simulink library "pixhawk_slib_adv"  (R2017b)
settings: Solver=ode45  StartTime=0.0  StopTime=10.0  RelTol=1e-3
undefined symbols (not defined in the file or in its folder): Earth, earthRadius, ModelInit_AngEuler, ModelInit_PosE, ModelInit_RateB, ModelInit_RPM, ModelInit_VelB, ModelParam_envAltitude, ModelParam_GPSLatLong, ModelParam_motorCr, ModelParam_motorJm, ModelParam_motorT, ModelParam_motorWb, ModelParam_noisePowerIMU, ModelParam_rotorCm, ModelParam_rotorCt, ModelParam_uavCCm, ModelParam_uavCd, ModelParam_uavDearo, ModelParam_uavJ, ModelParam_uavMass, ModelParam_uavR, ModelParam_uavType, Receive, Send, WGS84
libraries: etargetslib x11, dspnetwork x9, simulink x8, sharedtransform x5, aerolibtransform2 x4, aerolibutil x4, pixhawk_slib_adv x3, aerolibfltsims x3, shared6dof x1, aerolibobsolete x1, aerolibasang x1, aerolibatmos2 x1
(part 3 of 3)

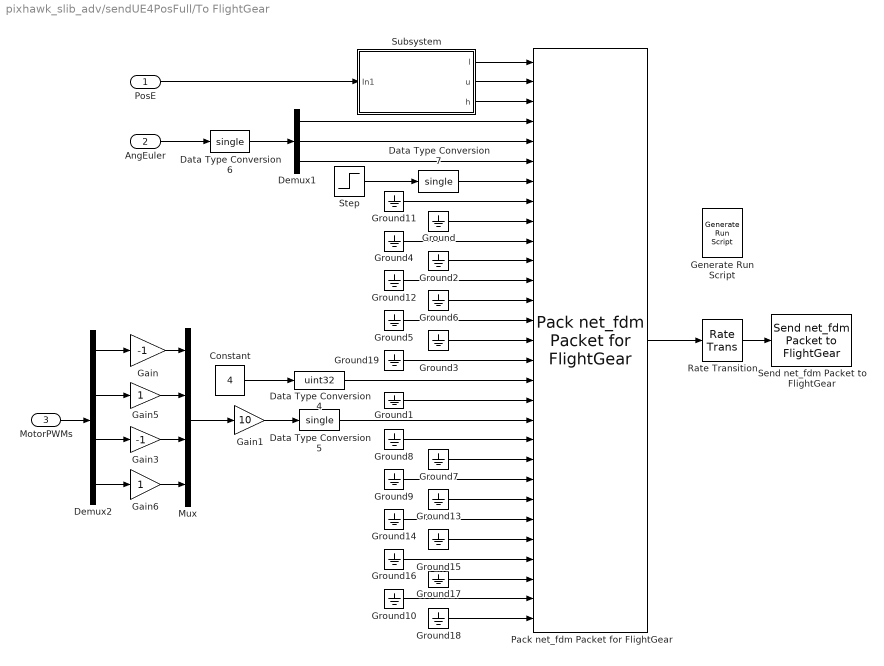
== system pixhawk_slib_adv/sendUE4PosFull/To FlightGear ==
  PosE : Inport
  AngEuler : Inport  Port=2
  MotorPWMs : Inport  Port=3
  Constant : Constant  Value=4
  Data Type Conversion4 : DataTypeConversion  OutDataTypeStr=uint32
  Data Type Conversion5 : DataTypeConversion  OutDataTypeStr=single
  Data Type Conversion6 : DataTypeConversion  OutDataTypeStr=single
  Data Type Conversion7 : DataTypeConversion  OutDataTypeStr=single
  Demux1 : Demux  Outputs=3
  Demux2 : Demux
  Gain : Gain  Gain=-1
  Gain1 : Gain  Gain=10
  Gain3 : Gain  Gain=-1
  Gain5 : Gain
  Gain6 : Gain
  Generate Run Script : aerolibfltsims/Generate Run Script  OutputFileName=runfg_myownUAV.bat  FlightGearBaseDirectory=C:\Program Files\FlightGear 2016.1.2  GeometryModelName=myownUAV  DestinationPort=5502  OriginAddress=127.0.0.1  OriginPort=5505  LocalAddress=127.0.0.1  AirportId=KSFO  RunwayId=10L  InitialAltitude=0  InitialHeading=0  OffsetDistance=0  OffsetAzimuth=0  GenerateFile=off  Architecture=Default  dataFlow=Send-Receive
  Ground{,1..19} (20 alike) : Ground
  Mux : Mux
  Pack net_fdm Packet for FlightGear : aerolibfltsims/Pack net_fdm Packet for FlightGear  FlightGearVersion=v2016.1  ShowPositionAttitudeInputs=on  ShowVelocityAccelerationInputs=off  ShowControlSurfacePositionInputs=on  ShowEngineFuelInputs=on  ShowLandingGearInputs=off  ShowEnvironmentInputs=off  SampleTime=0.01
      settings: SourceProductName=Aerospace Blockset  SourceProductBaseCode=AE
  Rate Transition : RateTransition
  Send net_fdm Packet to FlightGear : aerolibfltsims/Send net_fdm Packet to FlightGear  DestinationIpAddress=127.0.0.1  DestinationPort=5502  LocalIpPort=-1  varLen=off  SampleTime=0.005
      settings: SourceProductName=Aerospace Blockset  SourceProductBaseCode=AE
  Step : Step  Time=0  SampleTime=0
  Subsystem : Subsystem
  wires:
  Gain1/1 -> Data Type Conversion5/1
  Data Type Conversion6/1 -> Demux1/1
  Demux1/3 -> Pack net_fdm Packet for FlightGear/6
  Demux1/2 -> Pack net_fdm Packet for FlightGear/5
  Demux1/1 -> Pack net_fdm Packet for FlightGear/4
  Ground19/1 -> Pack net_fdm Packet for FlightGear/16
  Subsystem/3(h) -> Pack net_fdm Packet for FlightGear/3
  Subsystem/2(u) -> Pack net_fdm Packet for FlightGear/2
  Subsystem/1("l ") -> Pack net_fdm Packet for FlightGear/1
  PosE/1 -> Subsystem/1(In1)
  Rate Transition/1 -> Send net_fdm Packet to FlightGear/1
  Gain6/1 -> Mux/4
  Demux2/4 -> Gain6/1
  Gain5/1 -> Mux/2
  Demux2/2 -> Gain5/1
  Gain3/1 -> Mux/3
  Gain/1 -> Mux/1
  Demux2/3 -> Gain3/1
  Demux2/1 -> Gain/1
  Mux/1 -> Gain1/1
  MotorPWMs/1 -> Demux2/1
  AngEuler/1 -> Data Type Conversion6/1
  Ground12/1 -> Pack net_fdm Packet for FlightGear/12
  Ground2/1 -> Pack net_fdm Packet for FlightGear/11
  Data Type Conversion5/1 -> Pack net_fdm Packet for FlightGear/19
  Constant/1 -> Data Type Conversion4/1
  Ground11/1 -> Pack net_fdm Packet for FlightGear/8
  Ground4/1 -> Pack net_fdm Packet for FlightGear/10
  Ground6/1 -> Pack net_fdm Packet for FlightGear/13
  Ground5/1 -> Pack net_fdm Packet for FlightGear/14
  Ground3/1 -> Pack net_fdm Packet for FlightGear/15
  Ground1/1 -> Pack net_fdm Packet for FlightGear/18
  Data Type Conversion4/1 -> Pack net_fdm Packet for FlightGear/17
  Step/1 -> Data Type Conversion7/1
  Ground18/1 -> Pack net_fdm Packet for FlightGear/29
  Ground10/1 -> Pack net_fdm Packet for FlightGear/28
  Ground17/1 -> Pack net_fdm Packet for FlightGear/27
  Ground16/1 -> Pack net_fdm Packet for FlightGear/26
  Ground15/1 -> Pack net_fdm Packet for FlightGear/25
  Ground14/1 -> Pack net_fdm Packet for FlightGear/24
  Ground13/1 -> Pack net_fdm Packet for FlightGear/23
  Ground9/1 -> Pack net_fdm Packet for FlightGear/22
  Ground7/1 -> Pack net_fdm Packet for FlightGear/21
  Ground/1 -> Pack net_fdm Packet for FlightGear/9
  Ground8/1 -> Pack net_fdm Packet for FlightGear/20
  Data Type Conversion7/1 -> Pack net_fdm Packet for FlightGear/7
  Pack net_fdm Packet for FlightGear/1 -> Rate Transition/1

== system pixhawk_slib_adv/CopterMotorModel/MotorNonlinearDynamic1/Motor_Dynamics ==
  motor_rate_d : Inport
  ModelInit_RPM : Inport  Port=2
  motorT : Inport  Port=3
  Add : Sum  Inputs=+-
  Divide : Product  Inputs=*/
  Integrator : Integrator  InitialConditionSource=external
  motor_rate_act : Outport
  wires:
  motorT/1 -> Divide/2
  Integrator/1 -> Add/2, motor_rate_act/1  "x"
  Divide/1 -> Integrator/1  "drate/dt"
  motor_rate_d/1 -> Add/1
  ModelInit_RPM/1 -> Integrator/2
  Add/1 -> Divide/1

== system pixhawk_slib_adv/CopterMotorModel/MotorNonlinearDynamic2/Motor_Dynamics ==
  motor_rate_d : Inport
  ModelInit_RPM : Inport  Port=2
  motorT : Inport  Port=3
  Add : Sum  Inputs=+-
  Divide : Product  Inputs=*/
  Integrator : Integrator  InitialConditionSource=external
  motor_rate_act : Outport
  wires:
  Add/1 -> Divide/1
  ModelInit_RPM/1 -> Integrator/2
  motor_rate_d/1 -> Add/1
  Divide/1 -> Integrator/1  "drate/dt"
  Integrator/1 -> motor_rate_act/1, Add/2  "x"
  motorT/1 -> Divide/2

== system pixhawk_slib_adv/CopterMotorModel/MotorNonlinearDynamic3/Motor_Dynamics ==
  motor_rate_d : Inport
  ModelInit_RPM : Inport  Port=2
  motorT : Inport  Port=3
  Add : Sum  Inputs=+-
  Divide : Product  Inputs=*/
  Integrator : Integrator  InitialConditionSource=external
  motor_rate_act : Outport
  wires:
  motorT/1 -> Divide/2
  Integrator/1 -> Add/2, motor_rate_act/1  "x"
  Divide/1 -> Integrator/1  "drate/dt"
  motor_rate_d/1 -> Add/1
  ModelInit_RPM/1 -> Integrator/2
  Add/1 -> Divide/1

== system pixhawk_slib_adv/CopterMotorModel/MotorNonlinearDynamic4/Motor_Dynamics ==
  motor_rate_d : Inport
  ModelInit_RPM : Inport  Port=2
  motorT : Inport  Port=3
  Add : Sum  Inputs=+-
  Divide : Product  Inputs=*/
  Integrator : Integrator  InitialConditionSource=external
  motor_rate_act : Outport
  wires:
  Add/1 -> Divide/1
  ModelInit_RPM/1 -> Integrator/2
  motor_rate_d/1 -> Add/1
  Divide/1 -> Integrator/1  "drate/dt"
  Integrator/1 -> motor_rate_act/1, Add/2  "x"
  motorT/1 -> Divide/2

== system pixhawk_slib_adv/CopterMotorModel/MotorNonlinearDynamic5/Motor_Dynamics ==
  motor_rate_d : Inport
  ModelInit_RPM : Inport  Port=2
  motorT : Inport  Port=3
  Add : Sum  Inputs=+-
  Divide : Product  Inputs=*/
  Integrator : Integrator  InitialConditionSource=external
  motor_rate_act : Outport
  wires:
  motorT/1 -> Divide/2
  Integrator/1 -> Add/2, motor_rate_act/1  "x"
  Divide/1 -> Integrator/1  "drate/dt"
  motor_rate_d/1 -> Add/1
  ModelInit_RPM/1 -> Integrator/2
  Add/1 -> Divide/1

== system pixhawk_slib_adv/CopterMotorModel/MotorNonlinearDynamic6/Motor_Dynamics ==
  motor_rate_d : Inport
  ModelInit_RPM : Inport  Port=2
  motorT : Inport  Port=3
  Add : Sum  Inputs=+-
  Divide : Product  Inputs=*/
  Integrator : Integrator  InitialConditionSource=external
  motor_rate_act : Outport
  wires:
  Add/1 -> Divide/1
  ModelInit_RPM/1 -> Integrator/2
  motor_rate_d/1 -> Add/1
  Divide/1 -> Integrator/1  "drate/dt"
  Integrator/1 -> motor_rate_act/1, Add/2  "x"
  motorT/1 -> Divide/2

== system pixhawk_slib_adv/CopterMotorModel/MotorNonlinearDynamic7/Motor_Dynamics ==
  motor_rate_d : Inport
  ModelInit_RPM : Inport  Port=2
  motorT : Inport  Port=3
  Add : Sum  Inputs=+-
  Divide : Product  Inputs=*/
  Integrator : Integrator  InitialConditionSource=external
  motor_rate_act : Outport
  wires:
  motorT/1 -> Divide/2
  Integrator/1 -> Add/2, motor_rate_act/1  "x"
  Divide/1 -> Integrator/1  "drate/dt"
  motor_rate_d/1 -> Add/1
  ModelInit_RPM/1 -> Integrator/2
  Add/1 -> Divide/1

== system pixhawk_slib_adv/CopterMotorModel/MotorNonlinearDynamic8/Motor_Dynamics ==
  motor_rate_d : Inport
  ModelInit_RPM : Inport  Port=2
  motorT : Inport  Port=3
  Add : Sum  Inputs=+-
  Divide : Product  Inputs=*/
  Integrator : Integrator  InitialConditionSource=external
  motor_rate_act : Outport
  wires:
  Add/1 -> Divide/1
  ModelInit_RPM/1 -> Integrator/2
  motor_rate_d/1 -> Add/1
  Divide/1 -> Integrator/1  "drate/dt"
  Integrator/1 -> motor_rate_act/1, Add/2  "x"
  motorT/1 -> Divide/2

== system pixhawk_slib_adv/SensorOutput/HILGPSModel/GyroNoiseSwitch1 ==
  In1 : Inport
  Constant1 : Constant  Value=Param_GlobalNoiseGainSwitch
  Constant2 : Constant  Value=0.3
  Gain2 : Gain  Gain=0.7
  Product4 : Product
  Sum : Sum  Inputs=|++
  Out1 : Outport
  wires:
  Sum/1 -> Product4/2
  Product4/1 -> Out1/1
  Gain2/1 -> Sum/1
  In1/1 -> Product4/1
  Constant1/1 -> Gain2/1
  Constant2/1 -> Sum/2

== system pixhawk_slib_adv/SensorOutput/HILGPSModel/NoiseFilter1 ==
  In1 : Inport
  Demux : Demux  Outputs=3
  Mux1 : Mux  Inputs=3
  Transfer Fcn1 : TransferFcn  Denominator=[0.05 1]
  Transfer Fcn2 : TransferFcn  Denominator=[0.05 1]
  Transfer Fcn4 : TransferFcn  Denominator=[0.05 1]
  Out1 : Outport
  wires:
  Mux1/1 -> Out1/1
  In1/1 -> Demux/1
  Demux/3 -> Transfer Fcn2/1
  Transfer Fcn4/1 -> Mux1/1
  Transfer Fcn2/1 -> Mux1/3
  Demux/1 -> Transfer Fcn4/1
  Transfer Fcn1/1 -> Mux1/2
  Demux/2 -> Transfer Fcn1/1

== system pixhawk_slib_adv/SensorOutput/HILGPSModel/Subsystem ==
  u : Inport
  Constant : Constant  Value=0
  Constant1 : Constant  Value=360
  Demux1 : Demux  Outputs=3
  Product : Product
  Product1 : Product
  Sqrt : Sqrt  SaturateOnIntegerOverflow=on
  Sum1 : Sum  Inputs=|++
  Sum4 : Sum  Inputs=|++
  Switch : Switch  Threshold=1
  Switch1 : Switch
  Terminator : Terminator
  Trigonometric Function : Trigonometry  Operator=atan2
  v : Outport
  cot : Outport  Port=2
  wires:
  Demux1/2 -> Trigonometric Function/2, Product1/2, Product1/1
  Product/1 -> Sum4/1
  u/1 -> Demux1/1
  Switch/1 -> Sum1/1, Switch1/1, Switch1/2
  Product1/1 -> Sum4/2
  Demux1/3 -> Terminator/1
  Sqrt/1 -> v/1, Switch/2
  Constant/1 -> Switch/3
  Trigonometric Function/1 -> Switch/1
  Sum4/1 -> Sqrt/1
  Demux1/1 -> Trigonometric Function/1, Product/1, Product/2
  Constant1/1 -> Sum1/2
  Sum1/1 -> Switch1/3
  Switch1/1 -> cot/1

== system pixhawk_slib_adv/SensorOutput/HILSensorMavModel/GyroNoiseSwitch0 ==
  In1 : Inport
  Constant1 : Constant  Value=Param_GlobalNoiseGainSwitch
  Constant2 : Constant  Value=0.2
  Gain2 : Gain  Gain=0.8
  Product4 : Product
  Sum : Sum  Inputs=|++
  Out1 : Outport
  wires:
  Sum/1 -> Product4/2
  Product4/1 -> Out1/1
  Gain2/1 -> Sum/1
  In1/1 -> Product4/1
  Constant1/1 -> Gain2/1
  Constant2/1 -> Sum/2

== system pixhawk_slib_adv/SensorOutput/HILSensorMavModel/GyroNoiseSwitch1 ==
  In1 : Inport
  Constant1 : Constant  Value=Param_GlobalNoiseGainSwitch
  Constant2 : Constant  Value=0.2
  Gain2 : Gain  Gain=0.8
  Product4 : Product
  Sum : Sum  Inputs=|++
  Out1 : Outport
  wires:
  Sum/1 -> Product4/2
  Product4/1 -> Out1/1
  Gain2/1 -> Sum/1
  In1/1 -> Product4/1
  Constant1/1 -> Gain2/1
  Constant2/1 -> Sum/2

== system pixhawk_slib_adv/SensorOutput/HILSensorMavModel/GyroNoiseSwitch2 ==
  In1 : Inport
  Constant1 : Constant  Value=Param_GlobalNoiseGainSwitch
  Constant2 : Constant  Value=0.2
  Gain2 : Gain  Gain=0.8
  Product4 : Product
  Sum : Sum  Inputs=|++
  Out1 : Outport
  wires:
  Sum/1 -> Product4/2
  Product4/1 -> Out1/1
  Gain2/1 -> Sum/1
  In1/1 -> Product4/1
  Constant1/1 -> Gain2/1
  Constant2/1 -> Sum/2

== system pixhawk_slib_adv/SensorOutput/HILSensorMavModel/GyroNoiseSwitch3 ==
  In1 : Inport
  Constant1 : Constant  Value=Param_GlobalNoiseGainSwitch
  Constant2 : Constant  Value=0.3
  Gain2 : Gain  Gain=0.7
  Product4 : Product
  Sum : Sum  Inputs=|++
  Out1 : Outport
  wires:
  Sum/1 -> Product4/2
  Product4/1 -> Out1/1
  Gain2/1 -> Sum/1
  In1/1 -> Product4/1
  Constant1/1 -> Gain2/1
  Constant2/1 -> Sum/2

== system pixhawk_slib_adv/SensorOutput/HILSensorMavModel/GyroNoiseSwitch4 ==
  In1 : Inport
  Constant1 : Constant  Value=Param_GlobalNoiseGainSwitch
  Constant2 : Constant  Value=0.3
  Gain2 : Gain  Gain=0.7
  Product4 : Product
  Sum : Sum  Inputs=|++
  Out1 : Outport
  wires:
  Sum/1 -> Product4/2
  Product4/1 -> Out1/1
  Gain2/1 -> Sum/1
  In1/1 -> Product4/1
  Constant1/1 -> Gain2/1
  Constant2/1 -> Sum/2

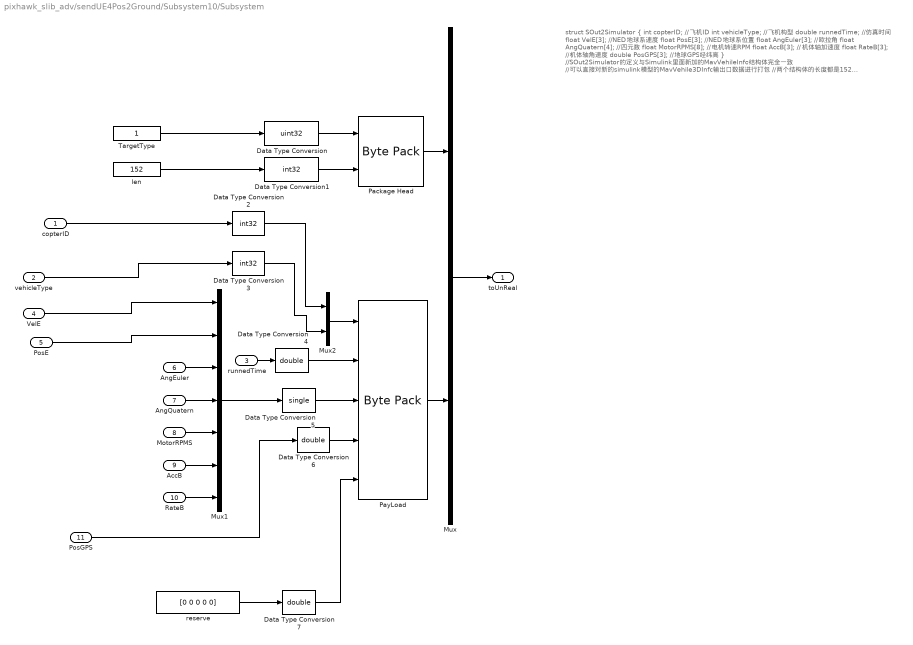
== system pixhawk_slib_adv/sendUE4Pos2Ground/Subsystem10/Subsystem ==
  note: struct SOut2Simulator
      | {
      | int copterID; //飞机ID
      | int vehicleType; //飞机构型
      | double runnedTime; //仿真时间
      | float VelE[3]; //NED地球系速度
      | float PosE[3]; //NED地球系位置
      | float AngEuler[3]; //欧拉角
      | float AngQuatern[4]; //四元数
      | float MotorRPMS[8]; //电机转速RPM
      | float AccB[3]; //机体轴加速度
      | float RateB[3]; //机体轴角速度
      | double PosGPS[3]; //地球GPS经纬高
      | }
      |
      | //SOut2Simulator的定义与Simulink里面新加的MavVehileInfo结构体完全一致
      | //可以直接对新的simulink模型的MavVehile3DInfo输出口数据进行打包
      | //两个结构体的长度都是152
      | sizeof(SOut2Simulator) = sizeof(MavVehileInfo) = 152
      |
      | 打包封装的结构体为
      | typedef struct _netDataShort
      | {
      | TargetType tg; //这里目前随便填，写1即可 uint32
      | int len; //这个长度为传输结构体长度，目前是152
      | char payload[192]; //这里面前152位存放了SOut2Simulator结构体数据，后面的40位保留
      | }netDataShort;
      |
      | //UDP包的总长度为200
      | sizeof(netDataShort) = 200
      |
      | //发送的UDP端口号为：20010
  copterID : Inport  PortDimensions=1
  vehicleType : Inport  Port=2  PortDimensions=1
  runnedTime : Inport  Port=3  PortDimensions=1
  "VelE " : Inport  Port=4  PortDimensions=3
  PosE : Inport  Port=5  PortDimensions=3
  AngEuler : Inport  Port=6  PortDimensions=3
  AngQuatern : Inport  Port=7  PortDimensions=4
  MotorRPMS : Inport  Port=8  PortDimensions=8
  AccB : Inport  Port=9  PortDimensions=3
  RateB : Inport  Port=10  PortDimensions=3
  PosGPS : Inport  Port=11  PortDimensions=3
  Data Type Conversion : DataTypeConversion  OutDataTypeStr=uint32
  Data Type Conversion1 : DataTypeConversion  OutDataTypeStr=int32
  Data Type Conversion2 : DataTypeConversion  OutDataTypeStr=int32
  Data Type Conversion3 : DataTypeConversion  OutDataTypeStr=int32
  Data Type Conversion4 : DataTypeConversion  OutDataTypeStr=double
  Data Type Conversion5 : DataTypeConversion  OutDataTypeStr=single
  Data Type Conversion6 : DataTypeConversion  OutDataTypeStr=double
  Data Type Conversion7 : DataTypeConversion  OutDataTypeStr=double
  Mux : Mux  Inputs=2
  Mux1 : Mux  Inputs=7
  Mux2 : Mux  Inputs=2
  Package Head : etargetslib/Byte Pack  datatypes={'uint32','int32'}  byteAlign=4
  PayLoad : etargetslib/Byte Pack  datatypes={'int32','double','single','double','double'}  byteAlign=8
  TargetType : Constant  OutDataTypeStr=Inherit: Inherit via back propagation
  len : Constant  Value=152  OutDataTypeStr=Inherit: Inherit via back propagation
  reserve : Constant  Value=[0 0 0 0 0]  OutDataTypeStr=double
  toUnReal : Outport
  wires:
  runnedTime/1 -> Data Type Conversion4/1
  RateB/1 -> Mux1/7
  PayLoad/1 -> Mux/2
  "VelE "/1 -> Mux1/1
  Mux1/1 -> Data Type Conversion5/1
  PosGPS/1 -> Data Type Conversion6/1
  Package Head/1 -> Mux/1
  AccB/1 -> Mux1/6
  Mux/1 -> toUnReal/1
  MotorRPMS/1 -> Mux1/5
  AngQuatern/1 -> Mux1/4
  copterID/1 -> Data Type Conversion2/1
  len/1 -> Data Type Conversion1/1
  vehicleType/1 -> Data Type Conversion3/1
  PosE/1 -> Mux1/2
  TargetType/1 -> Data Type Conversion/1
  reserve/1 -> Data Type Conversion7/1
  Mux2/1 -> PayLoad/1
  AngEuler/1 -> Mux1/3
  Data Type Conversion5/1 -> PayLoad/3
  Data Type Conversion2/1 -> Mux2/1
  Data Type Conversion1/1 -> Package Head/2
  Data Type Conversion6/1 -> PayLoad/4
  Data Type Conversion/1 -> Package Head/1
  Data Type Conversion3/1 -> Mux2/2
  Data Type Conversion4/1 -> PayLoad/2
  Data Type Conversion7/1 -> PayLoad/5

== system pixhawk_slib_adv/sendUE4PosFull/To FlightGear/Subsystem ==
  In1 : Inport
  Constant1 : Constant  Value=5  VectorParams1D=off
  Constant2 : Constant  Value=-2.1361  VectorParams1D=off
  Constant3 : Constant  Value=0.65673  VectorParams1D=off
  Demux : Demux  Outputs=3
  Gain1 : Gain  Gain=10/earthRadius
  Gain2 : Gain  Gain=10/earthRadius
  Gain4 : Gain
  Gain8 : Gain  Gain=-10
  Sum10 : Sum  Inputs=|++
  Sum8 : Sum  Inputs=|++
  Sum9 : Sum  Inputs=|++
  "l " : Outport
  u : Outport  Port=2
  h : Outport  Port=3
  wires:
  Sum8/1 -> "l "/1
  In1/1 -> Demux/1
  Sum9/1 -> u/1
  Sum10/1 -> h/1
  Gain4/1 -> Gain2/1
  Demux/2 -> Gain1/1
  Gain8/1 -> Sum10/1
  Gain1/1 -> Sum8/1
  Gain2/1 -> Sum9/1
  Constant2/1 -> Sum8/2
  Demux/3 -> Gain8/1
  Demux/1 -> Gain4/1
  Constant1/1 -> Sum10/2
  Constant3/1 -> Sum9/2

== matlab function pixhawk_slib_adv/getTerrainAltData ==
  data: x input; z output; y input
function z = fcn(x,y)
z=getTerrainAltData(x,y);

== matlab function pixhawk_slib_adv/CopterForceModel/Propeller Model old Version ==
  data: uavType input; MotorRads input; R input; Fb output; Mb output; Cm input; Ct input; Jm input; wb input
function [Fb,Mb] = fcn(uavType,MotorRads,R,Cm,Ct,Jm,wb)
% This is control effectiveness model, where Fb is the force produced by motors, Mb is
% the moment produced by motors, and Fd is the resistance produced by the air.
% The gyroscopic torque is not considered here.

% -1: anticlockwise, 1: clockwise 
TypeMotorDirMatrix=[...
    [-1 -1 -1 0 0 0 0 0];... % Tri 3*1 X
    [1 1 1 0 0 0 0 0];...    % Tri 3*1 +
    [-1 -1 1 1 0 0 0 0];... % Quad 4*1 X
    [-1 -1 1 1 0 0 0 0];... % Quad 4*1 +
    [1 -1 1 -1 -1 1 0 0];... % Hex 6*1 X
    [1 -1 1 -1 -1 1 0 0];... % Hex 6*1 +
    [1 -1 1 -1 1 -1 0 0];... % HexCoa 3*2
    [1 1 -1 -1 -1 -1 1 1];... % Oct 8*1 X
    [1 1 -1 -1 -1 -1 1 1];... % Oct 8*1 +
    [-1 1 -1 1 -1 1 -1 1];... % OctCoa 4*2 X
];

TypeMotorAngMatrix=[...
    [pi/3 pi -pi/3 0 0 0 0 0];...
    [pi/3 pi -pi/3 0 0 0 0 0];...
    [pi/4 pi/4+pi pi/4+3*pi/2 pi/4+pi/2 0 0 0 0];...
    [pi/2 3*pi/2 0 pi 0 0 0 0];...
    [pi/2 3/2*pi 3/2*pi+pi/3 pi/2+pi/3 pi/2-pi/3 3/2*pi-pi/3 0 0];...
    [0 pi pi+pi/3 pi/3 -pi/3 pi-pi/3 0 0];...
    [pi/3 pi/3 pi pi -pi/3 -pi/3 0 0];...
    [pi/8 pi+pi/8 pi/8+pi/4 pi-pi/8 -pi/8 3/2*pi-pi/8 3/2*pi+pi/8 pi/2+pi/8];...
    [0 pi pi/4 3/4*pi -pi/4 pi+pi/4 3/2*pi pi/2];...
    [pi/4 -pi/4 pi+pi/4 pi-pi/4 -pi/4 pi/4 pi-pi/4 pi+pi/4];...
];

TypeMotorNonVector=int8([3;3;4;4;6;6;6;8;8;8]);

Mb = [0;0;0];
Fb = [0;0;0];
P=wb(1);Q=wb(2);

if uavType==50
    
    Fb(1)=MotorRads(1)+MotorRads(3);
    Mb(3)=MotorRads(1)*0.1-MotorRads(3)*0.1;
    
    return;
end


if uavType<0||uavType>length(TypeMotorNonVector)
    uavType=int16(1);
end

TypeMotorDirVector=TypeMotorDirMatrix(uavType,:);
TypeMotorAngVector=TypeMotorAngMatrix(uavType,:);

for i=1:TypeMotorNonVector(uavType)
    propAng = TypeMotorAngVector(i);
    propdir = TypeMotorDirVector(i);
    PropT = Ct*MotorRads(i)*MotorRads(i);
    PropM = Cm*MotorRads(i)*MotorRads(i);
    
    %Thrust -> Moment
    Mb=Mb+[-R*sin(propAng)*PropT;R*cos(propAng)*PropT;-PropM*propdir];
    
    %gyroscopic moment
    Mb=Mb+[Q*Jm*MotorRads(i)*propdir;-P*Jm*MotorRads(i)*propdir;0];
    
    Fb=Fb+[0;0;-PropT];
end

 
end

== matlab function pixhawk_slib_adv/PlaneGroundModel/Ground Model ==
  settings: updateMethod=DISCRETE
  data: mg input; wb input; Xe input; F1 output; Ve input; M1 output; Quet input; terrainZ input
function [F1,M1] = fcn(mg,wb,Xe,Ve,Quet,terrainZ)
% This is a ground model that can provides reaction force and reaction torque

% persistent z0;
% if isempty(z0)
%      z0=0;
% end
terrainZ=terrainZ(1)
persistent takeoffFlag;
if isempty(takeoffFlag)
     takeoffFlag=int8(0);
end

persistent landFlag;
if isempty(landFlag)
     landFlag=int8(1);
end


z=Xe(3)-terrainZ;

 if (z<-0.3)&&(Ve(3)<-0.1)&&(takeoffFlag<0.5)
    takeoffFlag=int8(1);
    landFlag=int8(0);
 end
 
 if (z>-0.05)&&(Ve(3)>0.1)&&(landFlag<0.5)
    landFlag=int8(1);
    takeoffFlag=int8(0);
    %z0=terrainZ;
 end

takeoff = takeoffFlag;
landed = landFlag;


F1=[0;0;0];
M1=[0;0;0];

if z>=0
%     if z>=0.3
%         if Ve(3)>=5
%             F1(3)=-mg(3)-1000*Ve(3);
%         else
%             F1(3)=-mg(3)-500*z-100*Ve(3);  
%         end
%     elseif z>=0.1
%         if Ve(3)>=2
%             F1(3)=-mg(3)-100*Ve(3);
%         else
%             F1(3)=-mg(3)-50*z-100*Ve(3);  
%         end
%     else
%          if Ve(3)>=1
%             F1(3)=-mg(3)-50*Ve(3);
%         else
%             F1(3)=-mg(3)-5*z-50*Ve(3);  
%         end       
%     end
    if z<0.05
         F1(3)=-mg(3)-10*Ve(3); 
    elseif z<0.1
        F1(3)=-mg(3)-0.5*z-20*Ve(3); 
    else
         F1(3)=-mg(3)-1*z-50*Ve(3); 
    end

    
    F1(1)=-2*Ve(1);
    F1(2)=-50*Ve(2);
    M1=-20*[Quet(2);Quet(3);Quet(4)]-5*wb;
    M1 = M1 * abs(mg(3))*0.0333;
end

== matlab function pixhawk_slib_adv/LoadPngData ==
  data: pngMapName input
function fcn(pngMapName)

LoadPngData(pngMapName);

== matlab function pixhawk_slib_adv/CopterGroundModel/Ground Model ==
  settings: updateMethod=DISCRETE
  data: mg input; wb input; Xe input; F1 output; Ve input; M1 output; Quet input; TerrainIn input
function [F1,M1] = fcn(mg,wb,Xe,Ve,Quet,TerrainIn)
% This is a ground model that can provides reaction force and reaction torque

terrainZ=TerrainIn(1); %暂时提取高程数据

% persistent z0;
% if isempty(z0)
%      z0=0;
% end

persistent takeoffFlag;
if isempty(takeoffFlag)
     takeoffFlag=int8(0);
end

persistent landFlag;
if isempty(landFlag)
     landFlag=int8(1);
end


z=Xe(3)-terrainZ;

 if (z<-0.3)&&(Ve(3)<-0.1)&&(takeoffFlag<0.5)
    takeoffFlag=int8(1);
    landFlag=int8(0);
 end
 
 if (z>-0.05)&&(Ve(3)>0.1)&&(landFlag<0.5)
    landFlag=int8(1);
    takeoffFlag=int8(0);
    %z0=terrainZ;
 end

takeoff = takeoffFlag;
landed = landFlag;


F1=[0;0;0];
M1=[0;0;0];

if z>=0

    if z<0.01
         F1(3)=-mg(3)-200*z-200*Ve(3); 
    elseif z<0.03
        F1(3)=-mg(3)-500*z-500*Ve(3); 
    else
         F1(3)=-mg(3)-1000*z-1000*Ve(3); 
    end

    
    F1(1)=-50*Ve(1);
    F1(2)=-50*Ve(2);
    M1=-20*[Quet(2);Quet(3);Quet(4)]-5*wb;
    M1 = M1 * abs(mg(3))*0.0333;
end

== matlab function pixhawk_slib_adv/sendUE4CMD ==
  data: x input
function RflySendUE4CMD(x)
% x y z为设置相机的位置，单位m，北东地
%roll pitch yaw为设置相机方向，单位度

if ~exist('x','var')
   x='RflyChangeMapbyName Grasslands';
end

out = uint8(x);
len=length(out);
yy=[out,uint8(zeros(1,52-len))];
yy=[typecast(int32(1234567890),'uint8'),yy];
u=udp('255.255.255.255','RemotePort',20010);
fopen(u);
fwrite(u,yy);
fclose(u);
delete(u)

end

== matlab function pixhawk_slib_adv/RflyCameraPosAng ==
  data: x input; y input; z input; roll input; pitch input; yaw input
function RflyCameraPosAng(x,y,z,roll,pitch,yaw)
% x y z为设置相机的位置，单位m，北东地
%roll pitch yaw为设置相机方向，单位度

if ~exist('x','var')
   x=0;
end


if ~exist('y','var')
   y=0;
end

if ~exist('z','var')
   z=0;
end

if ~exist('roll','var')
   roll=0;
end

if ~exist('pitch','var')
   pitch=0;
end


if ~exist('yaw','var')
   yaw=0;
end

out = uint8(['RflyCameraPosAng ',num2str(x),' ',num2str(y),' ',num2str(z),' ',num2str(roll),' ',num2str(pitch),' ',num2str(yaw)]);
len=length(out);
yy=[out,uint8(zeros(1,52-len))];
yy=[typecast(int32(1234567890),'uint8'),yy];
u=udp('255.255.255.255','RemotePort',20010);
fopen(u);
fwrite(u,yy);
fclose(u);
delete(u)
%u3=udp('127.0.0.1','RemotePort',8848,'LocalPort',8850);%同上

end

== matlab function pixhawk_slib_adv/RflyChangeMap/MATLAB Function ==
  data: data output; input input
function data = ChangeMap(input)
    if ischar(input)
        % 通过地图名称修改
        cmd = ['RflyChangeMapbyName ', input];
    elseif isnumeric(input)
        % 通过地图ID修改
        cmd = ['RflyChangeMapbyID ', num2str(input)];
    else
        error('输入必须是字符串或数字');
    end
    
    % 将命令字符串转换为uint8并填充为252长度
    data = [uint8(cmd), uint8(zeros(1, 252 - length(cmd)))]; 
end

== matlab function pixhawk_slib_adv/SensorOutput/HILGPSModel/GenCogVel ==
  data: v output; u input; cot output
function [v,cot] = Ang360(u)
v=norm(u(1:2));

if v < 1
    cot = 0;
else
    cot=atan2d(u(2),u(1));
end
 
if cot<0
    cot=cot+360;
end

== matlab function pixhawk_slib_adv/sendUE4Pos2Ground/getTerrainAltData9 ==
  data: x input; z output; y input
function z = fcn(x,y)
z=getTerrainAltData(x,y);

== matlab function pixhawk_slib_adv/UDP_20100_PX4SilRecv/DataValidation ==
  data: inGPSPos input; outGPSPos output; inGpsVel input; inEulerAng input; outGpsVel output; outEulerAng output; outDataOk output
function [outGPSPos,outGpsVel,outEulerAng,outDataOk] = fcn(inGPSPos,inGpsVel,inEulerAng)

outGPSPos = [0;0;0];
outGpsVel = [0;0;0];
outEulerAng = [0;0;0];
outDataOk = 0;

if(abs(inGPSPos(1))<10000)
    outGPSPos=inGPSPos;
    outGpsVel=inGpsVel;
    outEulerAng = inEulerAng;
    outDataOk = 1;
end

== matlab function pixhawk_slib_adv/UDP_30100_TrueSimRecv/VehicleDataPerse1 ==
  data: Data input; y output double; dataOk output

% //FULL完整模式，输出到RflySim3D的数据
% struct SOut2Simulator {
%     int checksum; // 校验码123456789，必须设定为本值，才会认为是有效数据
%     int copterID;  //飞机ID序号
%     int vehicleType;  //载具样式ID，对应UE的XML中ClassID
%     int reserv; //备用标志位，Int型，将来用于表示碰撞、或大地图等标识
%     float VelE[3];   //速度，北东地，单位米/s
%     float AngEuler[3];  //欧拉角，滚转俯仰偏航，单位弧度
%     float AngQuatern[4]; //姿态四元数向量，w x y z
%     float MotorRPMS[8];  //执行器偏转量或转速，旋翼类对应RPM转每分
%     float AccB[3];       //载具机体FRD坐标系下加速度
%     float RateB[3];      //载具机体FRD坐标系下角速度，pqr，单位rad/s
%     double runnedTime; //时间戳，仿真开始为0时刻。
%     double PosE[3];   //北东地位置，单位米，z向下为正
%     double PosGPS[3];    //载具纬度、经度、高度向量，单位度和米，高度向上为正
% };
% // Python解码标识4i24f7d，数据长度168字节

% 
% 
% len = typecast(Data(5:8), 'int32');
% 
% if len ~= 152
%    return; 
% end
% 
% y = Data(9:160);
% dataOk = 1;

function [y, dataOk] = fcn(Data)
    % Initialize output
    dataOk = 0;

    % Persistent variable to store parsed data
    persistent UIV;
    if isempty(UIV)
        UIV = zeros(35, 1);
    end

    % Calculate length of the received data
    Length = numel(Data);

    % Check if data length matches the expected 168 bytes
    if Length == 168
        % Parse the checksum (first 4 bytes)
        checksum = typecast(Data(1:4), 'int32');
        
        % Verify checksum value
        if checksum == 123456789
            % Define index for parsing
            eIdx = 4 * 4;
            
            % Parse integer values (first 16 bytes)
            intVal = typecast(Data(1:eIdx), 'int32');
            
            % Parse single-precision float values (next 96 bytes)
            floatVal = typecast(Data(eIdx+1:eIdx+24*4), 'single');
            eIdx = eIdx + 24*4;
            
            % Parse double-precision float values (next 56 bytes)
            doubVal = typecast(Data(eIdx+1:eIdx+8*7), 'double');
            
            % Combine all parsed values into the persistent variable UIV
            UIV = [double(intVal); double(floatVal); doubVal];
            dataOk = 1;
        end
    end
    
    % Output the parsed data
    y = UIV;
end

== matlab function pixhawk_slib_adv/UDP_40100_RflyPx4Recv/VehicleDataPerse ==
  data: Data input; y output uint8 size=[48,1]; dataOk output
function [y, dataOk] = fcn(Data)
    % Initialize output
    y = uint8(zeros(48, 1));
    dataOk = 0;

    % Calculate length of the received data
    Length = numel(Data);

    % Check if data length matches the expected 48 bytes
    if Length ~= 48
        return;
    end

    % Parse the checksum (first 4 bytes)
    checksum = typecast(Data(1:4), 'int32');

    % Verify checksum value
    if checksum ~= 1234567898
        return;
    end

    % If checksum is correct, copy data to output
    y = Data(1:48);
    dataOk = 1;
end

== matlab function pixhawk_slib_adv/CopterForceModel/Body AeroCenter ==
  data: Fd output; Md output; wb input; Vb input; Cd input; CCm input; uavDearo input
function [Fd,Md] = fcn(wb,Vb,Cd, CCm, uavDearo)
% This is control effectiveness model, where Fb is the force produced by motors, Mb is
% the moment produced by motors, and Fd is the resistance produced by the air.
% The gyroscopic torque is not considered here.
% uavDearo 机身重心位置，向下为正

 Fd = -Cd*Vb.*abs(Vb);%
 
 Mfd=[Fd(2)*uavDearo;-Fd(1)*uavDearo;0];
 
Md=-CCm.*wb.*abs(wb);
Md=Mfd+Md;
%  CCm=4.72e-3;
%  Md=-CCm*wb.*abs(wb)*0.5;%0.3
%  Md= Mfd+Md;
 
end

== matlab function pixhawk_slib_adv/UDP_20100_PX4SilRecv/VehicleDataPerse ==
  data: Data input; y output uint8; dataOk output
function [y, dataOk] = fcn(Data)
    % Initialize output
    y = uint8(zeros(112, 1));
    dataOk = 0;

    % Calculate length of the received data
    Length = numel(Data);

    % Check if data length matches the expected 120 bytes
    if Length ~= 120
        return;
    end

    % Parse the length field from bytes 5 to 8
    len = typecast(Data(5:8), 'int32');

    % Verify parsed length
    if len ~= 112
        return;
    end

    % Extract the main data payload
    y = Data(9:120);
    dataOk = 1;
end
